simulink model "test"  (R2015a)
settings: Solver=ode5  StartTime=0.0  StopTime=10.0  FixedStep=1e-4  RelTol=1e-3
values from neighbouring files (symbols this model uses):
  Ak = [-64 -2560.5889522 8 186.2855092 1 -591.3291744 0 -1454.0827616 8 -3098.4577974 -142 -18500.7928836 ... (16 elements, 4x4)]    [controller.mat]    (also in main_matlab_step1.m = A-B*K-L*C)
  Ap = A(1:nn,1:nn)    [main_matlab_step1.m]    (also in plant.mat = [0 -330.46 0 -812.61 1 -12.15 0 -29.87 0 -2.44 0 -30.1 ... ()
  Bk = [64  -8; 2054  -280; -8  142; -1432  10169]    [controller.mat]    (also in main_matlab_step1.m = L)
  Bp = B    [main_matlab_step1.m]    (also in plant.mat = [0 2.71762 0 6.68268])
  Ck = [-64.81 -213.12 -1242.27 -85.82]    [controller.mat]    (also in main_matlab_step1.m = -K)
  Cp = C    [main_matlab_step1.m]    (also in plant.mat = [1  0  0  0; 0  0  1  0])
  Dk = [0 0]    [controller.mat]    (also in main_matlab_step1.m = zeros(1,2))
  GAMA1 = GAMA(1:naw,1:naw)    [main_matlab_step3.m]
  GAMA2 = GAMA(1:naw,naw+1:end)    [main_matlab_step3.m]
  GAMA3 = GAMA(naw+1:end,1:naw)    [main_matlab_step3.m]
  GAMA4 = GAMA(naw+1:end,naw+1:end)    [main_matlab_step3.m]
  Hp = H    [main_matlab_step1.m]    (also in plant.mat = [0 0 0 15.61])
  nc = 4    [find_N.m]    (also in main_matlab_step1.m = nk; main_matlab_step3.m = nn)
  nu = numel(Bpu)/np    [main_matlab_step1.m]    (also in main_matlab_step3.m = 1)
libraries: simulink x1
settings Model: Creator=p4wp4w  LastModifiedBy=p4wp4w

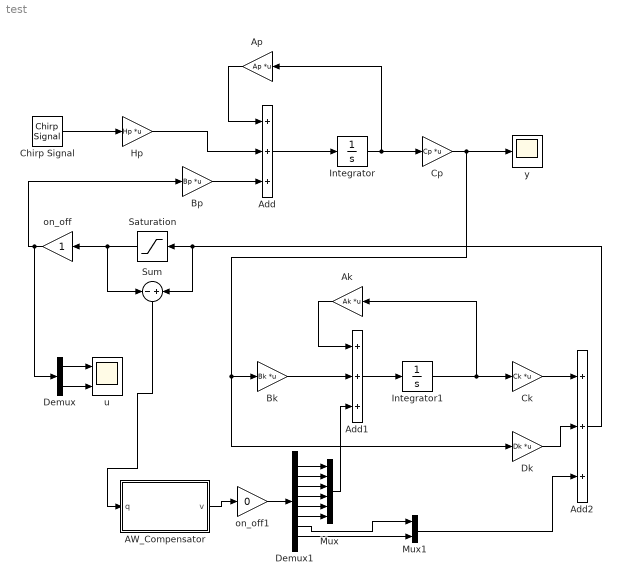
== system test ==
  AW_Compensator : Subsystem
  Add : Sum  Inputs=+++
  Add1 : Sum  Inputs=+++
  Add2 : Sum  Inputs=+++
  Ak : Gain  Gain=Ak  Multiplication=Matrix(K*u)
  Ap : Gain  Gain=Ap  Multiplication=Matrix(K*u)
  Bk : Gain  Gain=Bk  Multiplication=Matrix(K*u)
  Bp : Gain  Gain=Bp  Multiplication=Matrix(K*u)
  Chirp Signal : simulink/Sources/Chirp Signal  f1=0.1  T=14  f2=140
  Ck : Gain  Gain=Ck  Multiplication=Matrix(K*u)
  Cp : Gain  Gain=Cp  Multiplication=Matrix(K*u)
  Demux : Demux  Outputs=2
  Demux1 : Demux  Outputs=nc+nu
  Dk : Gain  Gain=Dk  Multiplication=Matrix(K*u)
  Hp : Gain  Gain=Hp  Multiplication=Matrix(K*u)
  Integrator : Integrator
  Integrator1 : Integrator
  Mux : Mux  Inputs=nc
  Mux1 : Mux  Inputs=nu
  Saturation : Saturate  UpperLimit=1.5  LowerLimit=-1.5
  Sum : Sum  Inputs=-|+
  on_off : Gain
  on_off1 : Gain  Gain=0
  u : Scope  NumInputPorts=2
      settings: YMin=-5~-5  YMax=5~5
  y : Scope
  wires:
  Add/1 -> Integrator/1
  Ap/1 -> Add/1
  Bp/1 -> Add/3
  Integrator/1 -> Cp/1, Ap/1
  Cp/1 -> Bk/1, Dk/1, y/1
  Hp/1 -> Add/2
  Chirp Signal/1 -> Hp/1
  on_off/1 -> Demux/1, Bp/1
  Add2/1 -> Sum/2, Saturation/1
  Demux/1 -> u/1
  Demux/2 -> u/2
  Saturation/1 -> Sum/1, on_off/1
  Add1/1 -> Integrator1/1
  Ak/1 -> Add1/1
  Integrator1/1 -> Ck/1, Ak/1
  Bk/1 -> Add1/2
  Ck/1 -> Add2/1
  Dk/1 -> Add2/2
  Sum/1 -> AW_Compensator/1(q)
  AW_Compensator/1(v) -> on_off1/1
  Demux1/1 -> Mux/1
  Demux1/2 -> Mux/2
  Demux1/3 -> Mux/3
  Demux1/4 -> Mux/4
  Demux1/5 -> Mux/5
  Demux1/6 -> Mux/6
  Demux1/7 -> Mux1/1
  Demux1/8 -> Mux1/2
  Mux1/1 -> Add2/3
  Mux/1 -> Add1/3
  on_off1/1 -> Demux1/1

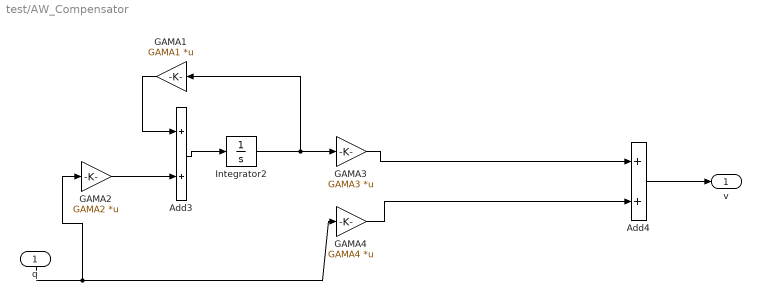
== system test/AW_Compensator ==
  q : Inport
  Add3 : Sum
  Add4 : Sum
  GAMA1 : Gain  Gain=GAMA1  Multiplication=Matrix(K*u)
  GAMA2 : Gain  Gain=GAMA2  Multiplication=Matrix(K*u)
  GAMA3 : Gain  Gain=GAMA3  Multiplication=Matrix(K*u)
  GAMA4 : Gain  Gain=GAMA4  Multiplication=Matrix(K*u)
  Integrator2 : Integrator
  v : Outport
  wires:
  Add3/1 -> Integrator2/1
  GAMA3/1 -> Add4/1
  q/1 -> GAMA2/1, GAMA4/1
  GAMA1/1 -> Add3/1
  Integrator2/1 -> GAMA3/1, GAMA1/1
  GAMA2/1 -> Add3/2
  GAMA4/1 -> Add4/2
  Add4/1 -> v/1
